simulink model "Part10"  (R2021a)
settings: Solver=VariableStepAuto  StartTime=0.0  StopTime=10.0  RelTol=1e-3
undefined symbols (not defined in the file): A, B, C, F, k, ka, L, T, x0
libraries: dspinverses x1
settings Model: Creator=ASUS  LastModifiedBy=ASUS

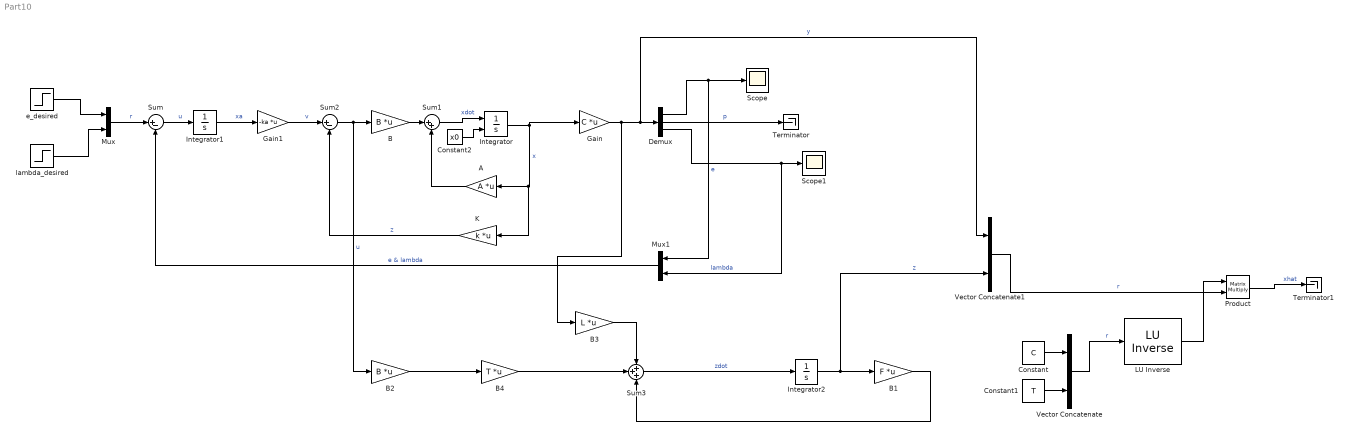
== system Part10 ==
  " LU Inverse" : dspinverses/ LU Inverse
  A : Gain  Gain=A  Multiplication=Matrix(K*u)
  B : Gain  Gain=B  Multiplication=Matrix(K*u)
  B1 : Gain  Gain=F  Multiplication=Matrix(K*u)
  B2 : Gain  Gain=B  Multiplication=Matrix(K*u)
  B3 : Gain  Gain=L  Multiplication=Matrix(K*u)
  B4 : Gain  Gain=T  Multiplication=Matrix(K*u)
  Constant : Constant  Value=C
  Constant1 : Constant  Value=T
  Constant2 : Constant  Value=x0
  Demux : Demux  Outputs=3
  Gain : Gain  Gain=C  Multiplication=Matrix(K*u)
  Gain1 : Gain  Gain=-ka  Multiplication=Matrix(K*u)
  Integrator : Integrator  InitialConditionSource=external
  Integrator1 : Integrator
  Integrator2 : Integrator
  K : Gain  Gain=k  Multiplication=Matrix(K*u)
  Mux : Mux  Inputs=2
  Mux1 : Mux  Inputs=2
  Product : Product  Multiplication=Matrix(*)
  Scope : Scope
  Scope1 : Scope
  Sum : Sum  Inputs=|+-
  Sum1 : Sum  Inputs=|++
  Sum2 : Sum  Inputs=|+-
  Sum3 : Sum  Inputs=+++
  Terminator : Terminator
  Terminator1 : Terminator
  Vector Concatenate : Concatenate  Mode=Multidimensional array
  Vector Concatenate1 : Concatenate  Mode=Multidimensional array
  e_desired : Step  Time=0  After=0.03  SampleTime=0
  lambda_desired : Step  Time=0  After=0.05  SampleTime=0
  wires:
  K/1 -> Sum2/2  "z"
  e_desired/1 -> Mux/1
  Demux/2 -> Terminator/1  "p"
  Integrator1/1 -> Gain1/1  "xa"
  Mux1/1 -> Sum/2  "e & lambda"
  lambda_desired/1 -> Mux/2
  Sum/1 -> Integrator1/1  "u"
  Sum2/1 -> B2/1, B/1  "u"
  Gain/1 -> Vector Concatenate1/1, Demux/1, B3/1  "y"
  Sum1/1 -> Integrator/1  "xdot"
  Gain1/1 -> Sum2/1  "v"
  A/1 -> Sum1/2
  Demux/1 -> Mux1/1, Scope/1  "e"
  B/1 -> Sum1/1
  Demux/3 -> Mux1/2, Scope1/1  "lambda"
  Mux/1 -> Sum/1  "r"
  Integrator/1 -> Gain/1, K/1, A/1  "x"
  Integrator2/1 -> Vector Concatenate1/2, B1/1  "z"
  B1/1 -> Sum3/3
  Sum3/1 -> Integrator2/1  "zdot"
  B3/1 -> Sum3/1
  Vector Concatenate1/1 -> Product/2  "r"
  Constant/1 -> Vector Concatenate/1
  Constant1/1 -> Vector Concatenate/2
  Vector Concatenate/1 -> " LU Inverse"/1  "r"
  " LU Inverse"/1 -> Product/1
  Product/1 -> Terminator1/1  "xhat"
  B4/1 -> Sum3/2
  B2/1 -> B4/1
  Constant2/1 -> Integrator/2
